simulink model "simulink_modelQ1_2"  (R2023a)
settings: Solver=FixedStepAuto  StartTime=0.0  StopTime=simulation_end_time  FixedStep=integration_step_time  RelTol=1e-3
values from neighbouring files (symbols this model uses):
  J_2 = 1.082e-3    (= 0.001082)    [main.m]
  myu = 398603    [main.m]
  r_0_vector = [-2.1 4.2 6.5]*10^3    [main.m]
  R_E = 6378    [main.m]
  v_0_vector = [-6.8 -1.5 -0.43]    [main.m]
settings Model: Creator=אלמוג  LastModifiedBy=אלמוג

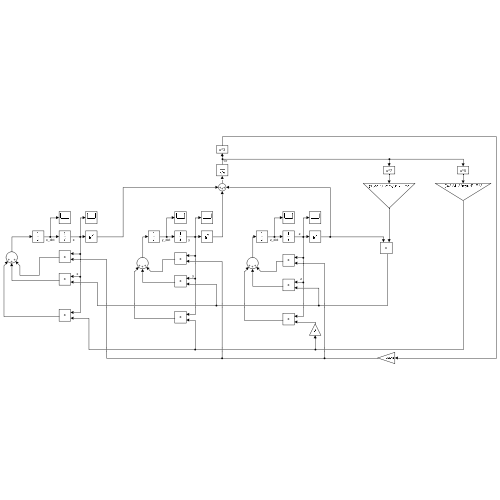
[thumbnail: Simulink's stored preview of the top-level diagram]
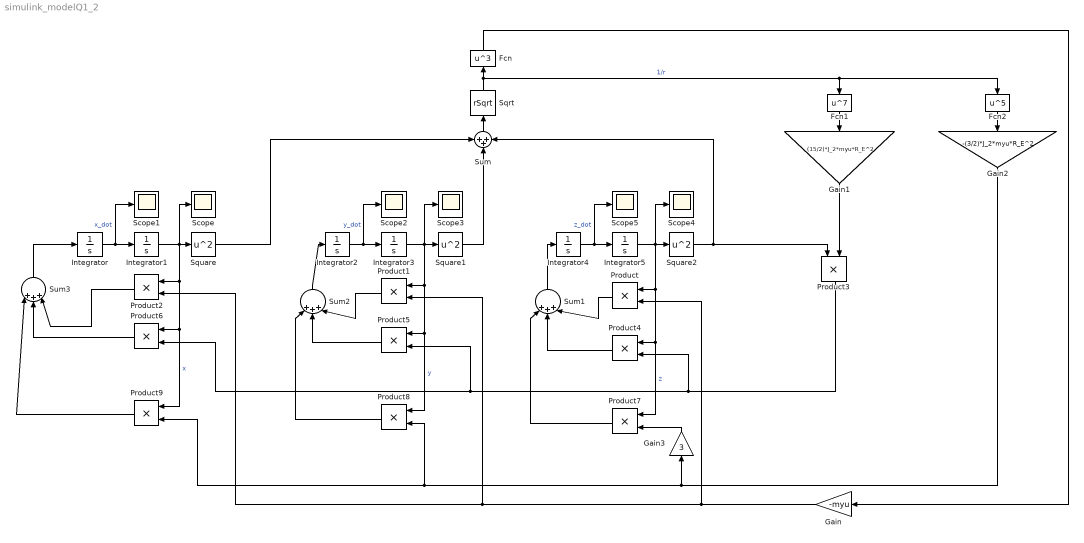
== system simulink_modelQ1_2 ==
  Fcn : Fcn  Expr=u^3
  Fcn1 : Fcn  Expr=u^7
  Fcn2 : Fcn  Expr=u^5
  Gain : Gain  Gain=-myu
  Gain1 : Gain  Gain=(15/2)*J_2*myu*R_E^2
  Gain2 : Gain  Gain=-(3/2)*J_2*myu*R_E^2
  Gain3 : Gain  Gain=3
  Integrator : Integrator  InitialCondition=v_0_vector(1)
  Integrator1 : Integrator  InitialCondition=r_0_vector(1)
  Integrator2 : Integrator  InitialCondition=v_0_vector(2)
  Integrator3 : Integrator  InitialCondition=r_0_vector(2)
  Integrator4 : Integrator  InitialCondition=v_0_vector(3)
  Integrator5 : Integrator  InitialCondition=r_0_vector(3)
  Product{,1..9} (10 alike) : Product
  Scope{,1..5} (6 alike) : Scope
  Sqrt : Sqrt  Operator=rSqrt
  Square : Math  Operator=square
  Square1 : Math  Operator=square
  Square2 : Math  Operator=square
  Sum : Sum  Inputs=+++
  Sum1 : Sum  Inputs=|+++|
  Sum2 : Sum  Inputs=|+++|
  Sum3 : Sum  Inputs=|+++|
  wires:
  Integrator2/1 -> Scope2/1, Integrator3/1  "y_dot"
  Integrator/1 -> Scope1/1, Integrator1/1  "x_dot"
  Integrator4/1 -> Scope5/1, Integrator5/1  "z_dot"
  Integrator1/1 -> Product9/1, Product6/1, Product2/1, Square/1, Scope/1  "x"
  Square/1 -> Sum/1
  Square2/1 -> Product3/1, Sum/3
  Square1/1 -> Sum/2
  Sum/1 -> Sqrt/1
  Sqrt/1 -> Fcn2/1, Fcn1/1, Fcn/1  "1/r"
  Fcn/1 -> Gain/1
  Product/1 -> Sum1/3
  Gain/1 -> Product2/2, Product1/2, Product/2
  Fcn1/1 -> Gain1/1
  Gain1/1 -> Product3/2
  Product3/1 -> Product6/2, Product5/2, Product4/2
  Integrator5/1 -> Product7/1, Product4/1, Product/1, Square2/1, Scope4/1  "z"
  Product4/1 -> Sum1/2
  Sum1/1 -> Integrator4/1
  Product5/1 -> Sum2/2
  Integrator3/1 -> Product8/1, Product5/1, Product1/1, Square1/1, Scope3/1  "y"
  Product1/1 -> Sum2/3
  Sum2/1 -> Integrator2/1
  Product2/1 -> Sum3/3
  Product6/1 -> Sum3/2
  Sum3/1 -> Integrator/1
  Fcn2/1 -> Gain2/1
  Gain2/1 -> Product8/2, Product9/2, Gain3/1
  Gain3/1 -> Product7/2
  Product7/1 -> Sum1/1
  Product8/1 -> Sum2/1
  Product9/1 -> Sum3/1
